simulink model "fcmClientSimulink_archer"  (R2021a)
settings: Solver=FixedStepDiscrete  StartTime=0.0  StopTime=time  FixedStep=1/120  RelTol=1e-3  EnableMultiTasking=on
undefined symbols (not defined in the file): sldrtexcb_modeswitch, Standard_Devices, time, UDP_Protocol
libraries: slrealtimeutilitieslib x2, sldrtlib x2
Description:
  | Packet Input/Output
  | 
  | The example model "sldrtex_packetio" shows how to transfer data through UDP
  | communication protocol using binary encoding. The model sends data
  | within one computer, from one UDP port to another. You can modify the
  | model to communicate between two computers by splitting this model
  | into its send and receive parts and running the models on two computers.
  | The yellow blocks are used to send the data, the blue blocks
  | are used to receive the data. Then, please enter the IP addresses of the two
  | computers into the appropriate fields in the Board Setup dialog.
  | 
  | How to run this model in Normal Mode:
  | 
  | 1) Double-click the orange button to switch to Normal Mode if needed.
  | 2) Start the real-time execution using Simulation->Run.
  | 
  | How to run this model in External Mode:
  | 
  | 1) Double-click the orange button to switch to External Mode if needed.
  | 2) Start the real-time execution using Simulation->Run. The model will automatically
  |    build, connect to Simulink in External Mode and start.
settings Model: SimulationMode=external  ExtModeTrigDuration=1001  Creator=The MathWorks, Inc.  LastModifiedBy=Maciej Zasuwa
settings SolverCC: AlgebraicLoopSolver=TrustRegion
settings DataIOCC: LimitDataPoints=on  SaveFormat=Array  ReturnWorkspaceOutputs=off
settings OptimizationCC: ExpressionDepthLimit=2147483647  InitFltsAndDblsToZero=on  EfficientMapNaN2IntZero=off  LifeSpan=inf
settings DebuggingCC: UnderspecifiedInitializationDetection=Classic  MergeDetectMultiDrivingBlocksExec=none  SolverPrmCheckMsg=warning  FcnCallInpInsideContextMsg=warning  AllowSymbolicDim=off  StateNameClashWarn=warning  SFUnexpectedBacktrackingDiag=warning  SFNoUnconditionalDefaultTransitionDiag=warning  SFExecutionAtInitializationDiag=none  SFMachineParentedDataDiag=warning  ArithmeticOperatorsInVariantConditions=warning
settings HardwareCC: TargetBitPerLong=64  TargetBitPerPointer=64  TargetBitPerSizeT=64  TargetBitPerPtrDiffT=64  TargetIntDivRoundTo=Zero  TargetEndianess=LittleEndian  TargetWordSize=64  TargetHWDeviceType=Intel->x86-64
settings ModelReferenceCC: PropagateSignalLabelsOutOfModel=off
settings SFSimCC: SimUseLocalCustomCode=off  CustomCodeUndefinedFunction=UseInterfaceOnly
settings RTWCC: Description=Simulink Desktop Real-Time  SystemTargetFile=sldrt.tlc  TemplateMakefile=sldrt.tmf  RTWUseLocalCustomCode=off  RTWCompilerOptimization=on
settings CodeAppCC: MaxIdLength=95  StateflowObjectComments=on
settings SimulinkDesktopRealTimeCC: TargetPreCompLibLocation=C:\Program Files\MATLAB\R2021a\toolbox\sldrt\lib\win64  TargetLangStandard=C89/C90 (ANSI)  SupportVariableSizeSignals=off
settings ConfigComp: CovMetricSettings=dw  CovSaveCumulativeToWorkspaceVar=on  CovSaveSingleToWorkspaceVar=on  CovExternalEMLEnable=off  CovSFcnEnable=off

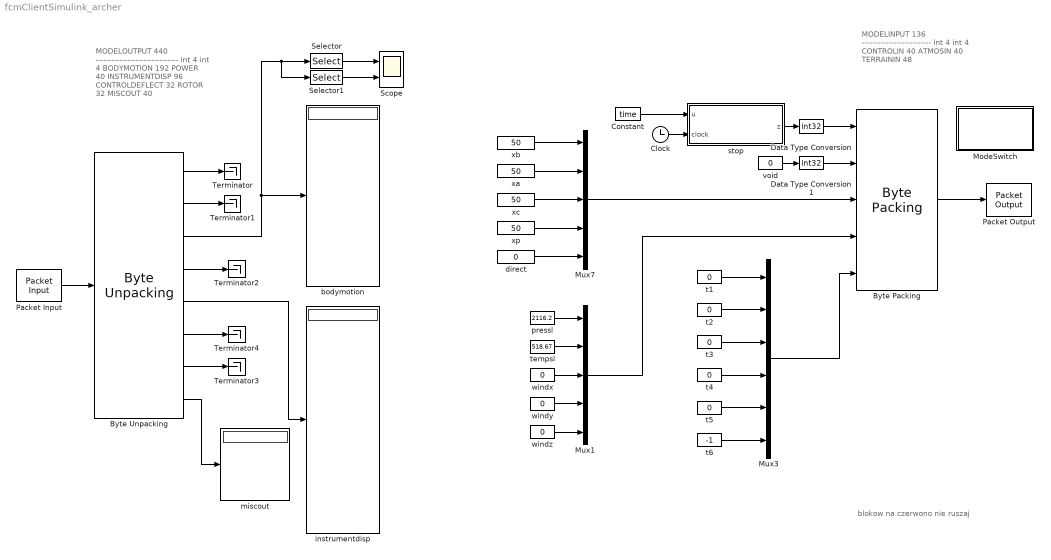
== system fcmClientSimulink_archer ==
  note: blokow na czerwono nie ruszaj
  note: MODELOUTPUT 440
      | -------------------------------
      | int 4
      | int 4
      | BODYMOTION 192
      | POWER 40
      | INSTRUMENTDISP 96
      | CONTROLDEFLECT 32
      | ROTOR 32
      | MISCOUT 40
  note: MODELINPUT  136
      | --------------------------
      | int 4
      | int 4
      | CONTROLIN  40
      | ATMOSIN  40
      | TERRAININ  48
  "Byte Packing " : slrealtimeutilitieslib/Byte Packing  MaskPackedDataType=uint8  MaskUnpackedDataTypes={'int32','int32','double','double','double'}  MaskAlignment=1
  "Byte Unpacking " : slrealtimeutilitieslib/Byte Unpacking  MaskUnpackedDataTypes={'int32','int32','double','double','double','double','double','double'}  MaskUnpackedDataSizes={[1] [1] [24] [5] [12] [4] [4] [5]}  MaskAlignment=1
      settings: SourceProductBaseCode=XP
  Clock : Clock
  Constant : Constant  Value=time
  Data Type Conversion : DataTypeConversion  OutDataTypeStr=int32  RndMeth=Nearest
  Data Type Conversion1 : DataTypeConversion  OutDataTypeStr=int32  RndMeth=Nearest
  ModeSwitch : Subsystem  InitFcn=sldrtexcb_modeswitch('CheckKernel');  mask(Simulink Desktop Real-Time Example Mode Switch){}
      settings: OpenFcn=sldrtexcb_modeswitch(gcbh);
      mask Display: disp('Switch To\nNormal Mode');
  Mux1 : Mux  Inputs=5
  Mux3 : Mux  Inputs=6
  Mux7 : Mux  Inputs=5
  Packet Input : sldrtlib/Packet Input  SampleTime=1/120  MaxMissedTicks=50  ShowMissedTicks=off  YieldWhenWaiting=off  DrvName=Standard_Devices/UDP_Protocol  DrvAddress=7101  DrvOptions=[2887123568 7101]  PacketSize=440  DataTypes={'440*uint8'}  ShowReady=off  ShowError=off  PacketID=1  ByteOrder=1  ShowTimestamp=off
      settings: AttributesFormatString=UDP Protocol [7101]
  Packet Output : sldrtlib/Packet Output  SampleTime=1/120  MaxMissedTicks=50  ShowMissedTicks=off  YieldWhenWaiting=off  DrvName=Standard_Devices/UDP_Protocol  DrvAddress=36864  DrvOptions=[2887123568 7100]  PacketSize=136  DataTypes={'136*uint8'}  ShowReady=off  ShowError=off  PacketID=1  ByteOrder=1  InitialValue=[]  FinalValue=[]
      settings: AttributesFormatString=UDP Protocol [36864]
  Scope : Scope  NumInputPorts=2
  Selector : Selector  InputPortWidth=24  IndexOptions=Index vector (dialog)  Indices=[1 2 3]  OutputSizes=1
  Selector1 : Selector  InputPortWidth=24  IndexOptions=Index vector (dialog)  Indices=[4 5 6]  OutputSizes=1
  Terminator{,1..4} (5 alike) : Terminator
  bodymotion : Display
  direct : Constant  Value=0  OutDataTypeStr=double  LockScale=on
  instrumentdisp : Display
  miscout : Display
  pressl : Constant  Value=2116.2  OutDataTypeStr=double  LockScale=on
  stop : MATLAB Function  TreatAsAtomicUnit=on  VariantControl=Variant1
  t{1..5} (5 alike) : Constant  Value=0  OutDataTypeStr=double  LockScale=on
  t6 : Constant  Value=-1  OutDataTypeStr=double  LockScale=on
  tempsl : Constant  Value=518.67  OutDataTypeStr=double  LockScale=on
  void : Constant  Value=0  OutDataTypeStr=double  LockScale=on
  windx : Constant  Value=0  OutDataTypeStr=double  LockScale=on
  windy : Constant  Value=0  OutDataTypeStr=double  LockScale=on
  windz : Constant  Value=0  OutDataTypeStr=double  LockScale=on
  xa : Constant  Value=50  OutDataTypeStr=double  LockScale=on
  xb : Constant  Value=50  OutDataTypeStr=double  LockScale=on
  xc : Constant  Value=50  OutDataTypeStr=double  LockScale=on
  xp : Constant  Value=50  OutDataTypeStr=double  LockScale=on
  wires:
  stop/1(z) -> Data Type Conversion/1
  "Byte Packing "/1 -> Packet Output/1
  Packet Input/1 -> "Byte Unpacking "/1
  Clock/1 -> stop/2(clock)
  Constant/1 -> stop/1(u)
  "Byte Unpacking "/2 -> Terminator1/1
  "Byte Unpacking "/1 -> Terminator/1
  "Byte Unpacking "/3 -> Selector1/1, Selector/1, bodymotion/1
  "Byte Unpacking "/4 -> Terminator2/1
  "Byte Unpacking "/5 -> instrumentdisp/1
  Mux7/1 -> "Byte Packing "/3
  xb/1 -> Mux7/1
  xa/1 -> Mux7/2
  xc/1 -> Mux7/3
  t5/1 -> Mux3/5
  t6/1 -> Mux3/6
  t1/1 -> Mux3/1
  t2/1 -> Mux3/2
  t3/1 -> Mux3/3
  t4/1 -> Mux3/4
  Mux3/1 -> "Byte Packing "/5
  Data Type Conversion/1 -> "Byte Packing "/1
  void/1 -> Data Type Conversion1/1
  Data Type Conversion1/1 -> "Byte Packing "/2
  Selector/1 -> Scope/1
  Selector1/1 -> Scope/2
  xp/1 -> Mux7/4
  "Byte Unpacking "/6 -> Terminator4/1
  direct/1 -> Mux7/5
  windy/1 -> Mux1/4
  windz/1 -> Mux1/5
  windx/1 -> Mux1/3
  pressl/1 -> Mux1/1
  tempsl/1 -> Mux1/2
  "Byte Unpacking "/7 -> Terminator3/1
  "Byte Unpacking "/8 -> miscout/1
  Mux1/1 -> "Byte Packing "/4

== system fcmClientSimulink_archer/ModeSwitch ==

== matlab function fcmClientSimulink_archer/stop ==
  data: u input; z output; clock input
function z     = stopControl (u, clock)

if clock >= (u-0.01)
    z = 0;
else
    z = 1;
end

end
